simulink model "test_link_demux"  (Simulink 7.3)
settings: Solver=ode45  StartTime=0.0  StopTime=300  RelTol=1e-3
libraries: xbsIndex_r4 x118, xps_library x6, isi_correlator_lib x6, casper_library x2
settings Model: Creator=wjm  LastModifiedBy=wjm
settings OptimizationCC: InitFltsAndDblsToZero=on

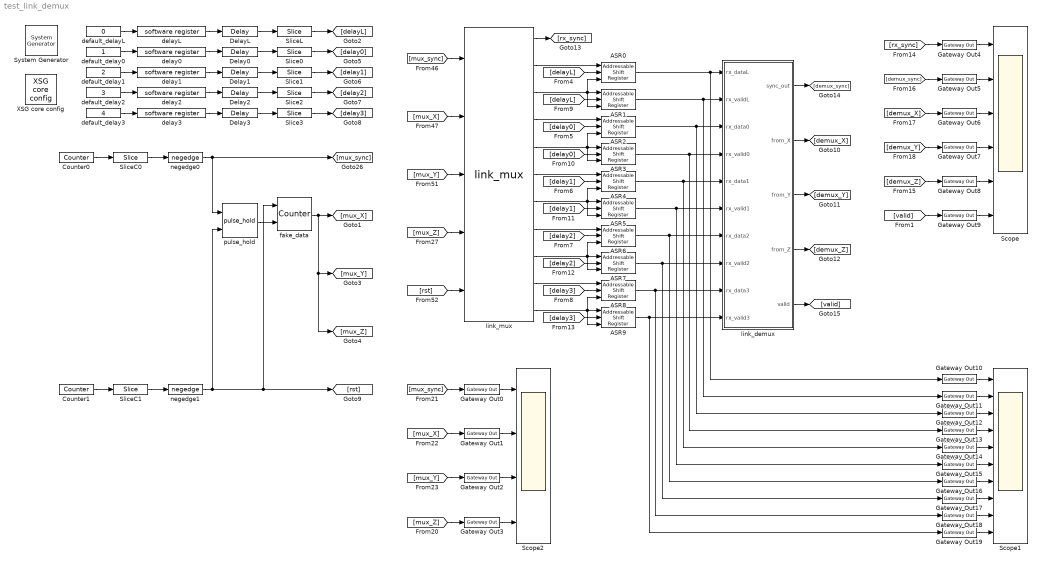
== system test_link_demux ==
  " System Generator" : xbsIndex_r4/ System Generator  Tag=genX  SystemSampleTime=-1  xilinxfamily=virtex5  part=xc5vsx95t  speed=-1  package=ff1136  synthesis_tool=XST  clock_wrapper=Clock Enables  directory=./isi_correlator_cropped/sysgen  testbench=off  simulink_period=1  sysclk_period=5  dcm_input_clock_period=100  incr_netlist=off  trim_vbits=Everywhere in SubSystem  dbl_ovrd=According to Block Masks  core_generation=According to Block Masks  run_coregen=off  deprecated_control=off  eval_field=0  block_type=sysgen
      settings: block_version=10.1.1
  ASR{0..9} (10 alike) : xbsIndex_r4/Addressable Shift Register  infer_latency=on  depth=2  initVector=[0]  en=on  dbl_ovrd=off  use_behavioral_HDL=off  use_rpm=off  block_type=addrsr
      settings: infoedit="Delay of configurable length.  Any element in the delay line can be addressed and driven onto the output port.<br><br>Hardware notes: This block is implemented using SRL16s. If Virtex-4 or Spartan-3 device is used, multiple SRLC16s are cascaded together."  block_version=10.1.3
  Counter0 : xbsIndex_r4/Counter  cnt_type=Free Running  cnt_to=Inf  operation=Up  start_count=2^7-1  cnt_by_val=1  arith_type=Unsigned  n_bits=7  bin_pt=0  load_pin=off  rst=off  en=off  explicit_period=on  period=1  dbl_ovrd=off  use_behavioral_HDL=off  implementation=Fabric  use_rpm=off  block_type=counter
  Counter1 : xbsIndex_r4/Counter  cnt_type=Free Running  cnt_to=Inf  operation=Up  start_count=2^7-1+5  cnt_by_val=1  arith_type=Unsigned  n_bits=9  bin_pt=0  load_pin=off  rst=off  en=off  explicit_period=on  period=1  dbl_ovrd=off  use_behavioral_HDL=off  implementation=Fabric  use_rpm=off  block_type=counter
  Delay{0..3} (4 alike) : xbsIndex_r4/Delay  en=off  latency=3  dbl_ovrd=off  reg_retiming=off  block_type=delay
  DelayL : xbsIndex_r4/Delay  en=off  latency=3  dbl_ovrd=off  reg_retiming=off  block_type=delay
  Gateway Out{0..19} (20 alike) : xbsIndex_r4/Gateway Out  hdl_port=on  timing_constraint=None  locs_specified=off  LOCs={}  block_type=gatewayout
      settings: infoedit="Gateway out block.  Converts Xilinx fixed point inputs into ouputs of type Simulink integer, double, or fixed point.<br><br>Hardware notes:  In hardware these blocks become top level output ports or are discarded, depending on how they are configured."  block_version=11.3
  Scope : Scope  NumInputPorts=6
      settings: TimeRange=150  YMin=0~-1~-1~-1~-1~-1  YMax=1~1~1~1~1~1
  Scope1 : Scope  NumInputPorts=10
      settings: YMin=-5~-5~-5~-5~-5~-5~-5~-5~-5~-5  YMax=5~5~5~5~5~5~5~5~5~5
  Scope2 : Scope  NumInputPorts=4
      settings: YMin=-5~-5~-5~-5  YMax=5~5~5~5  SaveName=ScopeData2
  Slice{0..3} (4 alike) : xbsIndex_r4/Slice  nbits=8  boolean_output=off  mode=Lower Bit Location + Width  bit1=0  base1=MSB of Input  bit0=0  base0=LSB of Input  dbl_ovrd=off  block_type=slice
      settings: block_version=10.1.3
  SliceC0 : xbsIndex_r4/Slice  nbits=1  boolean_output=on  mode=Upper Bit Location + Width  bit1=0  base1=MSB of Input  bit0=0  base0=LSB of Input  dbl_ovrd=off  block_type=slice
      settings: infoedit="Extracts a given range of bits from each input sample and presents it at the output.  The output type is ordinarily unsigned with binary point at zero, but can be Boolean when the slice is one bit wide.<P><P>Hardware notes: In hardware this block costs nothing."  block_version=10.1.3
  SliceC1 : xbsIndex_r4/Slice  nbits=1  boolean_output=on  mode=Upper Bit Location + Width  bit1=0  base1=MSB of Input  bit0=0  base0=LSB of Input  dbl_ovrd=off  block_type=slice
      settings: infoedit="Extracts a given range of bits from each input sample and presents it at the output.  The output type is ordinarily unsigned with binary point at zero, but can be Boolean when the slice is one bit wide.<P><P>Hardware notes: In hardware this block costs nothing."  block_version=10.1.3
  SliceL : xbsIndex_r4/Slice  nbits=8  boolean_output=off  mode=Lower Bit Location + Width  bit1=0  base1=MSB of Input  bit0=0  base0=LSB of Input  dbl_ovrd=off  block_type=slice
      settings: block_version=10.1.3
  XSG core config : xps_library/XSG core config  Tag=xps:xsg  SystemSampleTime=-1  hw_sys=ROACH:sx95t  ibob_linux=off  clk_src=adc0_clk  iBOB_clk_src=sys_clk  BEE2_ctrl_clk_src=sys_clk  BEE2_usr_clk_src=sys_clk  ROACH_clk_src=adc0_clk  CORR_clk_src=sys_clk  gpio_clk_io_group=iBOB:sma  gpio_clk_bit_index=0  clk_rate=200  sample_period=1  synthesis_tool=XST  mpc_type=powerpc440_ext
  default_delay0 : Constant  OutDataType=sfix(16)  OutScaling=2^0  SampleTime=1
  default_delay1 : Constant  Value=2  OutDataType=sfix(16)  OutScaling=2^0  SampleTime=1
  default_delay2 : Constant  Value=3  OutDataType=sfix(16)  OutScaling=2^0  SampleTime=1
  default_delay3 : Constant  Value=4  OutDataType=sfix(16)  OutScaling=2^0  SampleTime=1
  default_delayL : Constant  Value=0  OutDataType=sfix(16)  OutScaling=2^0  SampleTime=1
  delay0 : xps_library/software register  Tag=xps:sw_reg  SystemSampleTime=-1  io_dir=From Processor  arith_type=Unsigned  bitwidth=32  bin_pt=0  sample_period=1  gw_name=test_link_demux_delay0_user_data_out
      link override convert: arith_type=Unsigned  n_bits=32  bin_pt=0
      link override test_link_demux_delay0_user_data_out: arith_type=Unsigned  n_bits=32  bin_pt=0  period=1
  delay1 : xps_library/software register  Tag=xps:sw_reg  SystemSampleTime=-1  io_dir=From Processor  arith_type=Unsigned  bitwidth=32  bin_pt=0  sample_period=1  gw_name=test_link_demux_delay1_user_data_out
      link override convert: arith_type=Unsigned  n_bits=32  bin_pt=0
      link override test_link_demux_delay1_user_data_out: arith_type=Unsigned  n_bits=32  bin_pt=0  period=1
  delay2 : xps_library/software register  Tag=xps:sw_reg  SystemSampleTime=-1  io_dir=From Processor  arith_type=Unsigned  bitwidth=32  bin_pt=0  sample_period=1  gw_name=test_link_demux_delay2_user_data_out
      link override convert: arith_type=Unsigned  n_bits=32  bin_pt=0
      link override test_link_demux_delay2_user_data_out: arith_type=Unsigned  n_bits=32  bin_pt=0  period=1
  delay3 : xps_library/software register  Tag=xps:sw_reg  SystemSampleTime=-1  io_dir=From Processor  arith_type=Unsigned  bitwidth=32  bin_pt=0  sample_period=1  gw_name=test_link_demux_delay3_user_data_out
      link override convert: arith_type=Unsigned  n_bits=32  bin_pt=0
      link override test_link_demux_delay3_user_data_out: arith_type=Unsigned  n_bits=32  bin_pt=0  period=1
  delayL : xps_library/software register  Tag=xps:sw_reg  SystemSampleTime=-1  io_dir=From Processor  arith_type=Unsigned  bitwidth=32  bin_pt=0  sample_period=1  gw_name=test_link_demux_delayL_user_data_out
      link override convert: arith_type=Unsigned  n_bits=32  bin_pt=0
      link override test_link_demux_delayL_user_data_out: arith_type=Unsigned  n_bits=32  bin_pt=0  period=1
  fake_data : xbsIndex_r4/Counter  cnt_type=Free Running  cnt_to=Inf  operation=Up  start_count=0  cnt_by_val=1  arith_type=Unsigned  n_bits=30  bin_pt=0  load_pin=off  rst=on  en=on  explicit_period=on  period=1  dbl_ovrd=off  use_behavioral_HDL=off  implementation=Fabric  use_rpm=off  block_type=counter
  link_demux : Subsystem  AncestorBlock=isi_correlator_lib/link_demux  mask(link_demux){buffer_depth=8, logic_latency=1, mux_latency=1}
      mask prompts: buffer_depth "Buffer depth: (2^n)"; logic_latency "Logic latency:"; mux_latency "Mux latency:"
      mask help: Demuxes three data streams from five links (one loopback and four xaui). Realigns the streams, and reconstructs a corresponding sync pulse.
  link_mux : isi_correlator_lib/link_mux  SystemSampleTime=-1
  negedge0 : casper_library/Misc/negedge  Tag=Rising Edge Detector  SystemSampleTime=-1
  negedge1 : casper_library/Misc/negedge  Tag=Rising Edge Detector  SystemSampleTime=-1
  pulse_hold : isi_correlator_lib/pulse_hold  SystemSampleTime=-1
  wires:
  SliceC0/1 -> negedge0/1
  Counter0/1 -> SliceC0/1
  fake_data/1 -> [mux_Y], [mux_Z], [mux_X]
  SliceC1/1 -> negedge1/1
  Counter1/1 -> SliceC1/1
  negedge0/1 -> pulse_hold/1, [mux_sync]
  negedge1/1 -> pulse_hold/2, fake_data/1, [rst]
  pulse_hold/1 -> fake_data/2
  default_delayL/1 -> delayL/1
  delayL/1 -> DelayL/1
  default_delay0/1 -> delay0/1
  delay0/1 -> Delay0/1
  default_delay1/1 -> delay1/1
  delay1/1 -> Delay1/1
  default_delay2/1 -> delay2/1
  delay2/1 -> Delay2/1
  default_delay3/1 -> delay3/1
  delay3/1 -> Delay3/1
  DelayL/1 -> SliceL/1
  Delay0/1 -> Slice0/1
  Delay1/1 -> Slice1/1
  Delay2/1 -> Slice2/1
  Delay3/1 -> Slice3/1
  ASR0/1 -> link_demux/1(rx_dataL), Gateway Out10/1
  ASR1/1 -> link_demux/2(rx_validL), Gateway Out11/1
  ASR2/1 -> link_demux/3(rx_data0), Gateway Out12/1
  ASR3/1 -> link_demux/4(rx_valid0), Gateway Out13/1
  ASR4/1 -> link_demux/5(rx_data1), Gateway Out14/1
  ASR5/1 -> link_demux/6(rx_valid1), Gateway Out15/1
  ASR6/1 -> link_demux/7(rx_data2), Gateway Out16/1
  ASR7/1 -> link_demux/8(rx_valid2), Gateway Out17/1
  ASR8/1 -> link_demux/9(rx_data3), Gateway Out18/1
  ASR9/1 -> link_demux/10(rx_valid3), Gateway Out19/1
  link_mux/2 -> ASR0/1
  link_mux/3 -> ASR1/1, ASR0/3, ASR1/3
  link_mux/4 -> ASR2/1
  link_mux/5 -> ASR3/1, ASR2/3, ASR3/3
  link_mux/6 -> ASR4/1
  link_mux/7 -> ASR5/1, ASR4/3, ASR5/3
  link_mux/8 -> ASR6/1
  link_mux/9 -> ASR7/1, ASR6/3, ASR7/3
  link_mux/10 -> ASR8/1
  link_mux/11 -> ASR9/1, ASR8/3, ASR9/3
  [mux_sync] -> link_mux/1
  [mux_X] -> link_mux/2
  [mux_Y] -> link_mux/3
  [mux_Z] -> link_mux/4
  [rst] -> link_mux/5
  [delayL] -> ASR0/2
  [delayL] -> ASR1/2
  [delay0] -> ASR2/2
  [delay0] -> ASR3/2
  [delay1] -> ASR4/2
  [delay1] -> ASR5/2
  [delay2] -> ASR6/2
  [delay2] -> ASR7/2
  [delay3] -> ASR8/2
  [delay3] -> ASR9/2
  link_mux/1 -> [rx_sync]
  [rx_sync] -> Gateway Out4/1
  [demux_sync] -> Gateway Out5/1
  [demux_X] -> Gateway Out6/1
  [demux_Y] -> Gateway Out7/1
  [demux_Z] -> Gateway Out8/1
  [mux_sync] -> Gateway Out0/1
  [mux_X] -> Gateway Out1/1
  [mux_Y] -> Gateway Out2/1
  [mux_Z] -> Gateway Out3/1
  link_demux/1(sync_out) -> [demux_sync]
  link_demux/2(from_X) -> [demux_X]
  link_demux/3(from_Y) -> [demux_Y]
  link_demux/4(from_Z) -> [demux_Z]
  link_demux/5(valid) -> [valid]
  SliceL/1 -> [delayL]
  Slice0/1 -> [delay0]
  Slice1/1 -> [delay1]
  Slice2/1 -> [delay2]
  Slice3/1 -> [delay3]
  Gateway Out0/1 -> Scope2/1
  Gateway Out1/1 -> Scope2/2
  Gateway Out2/1 -> Scope2/3
  Gateway Out3/1 -> Scope2/4
  Gateway Out4/1 -> Scope/1
  Gateway Out5/1 -> Scope/2
  Gateway Out6/1 -> Scope/3
  Gateway Out7/1 -> Scope/4
  Gateway Out8/1 -> Scope/5
  Gateway Out10/1 -> Scope1/1
  Gateway Out11/1 -> Scope1/2
  Gateway Out12/1 -> Scope1/3
  Gateway Out13/1 -> Scope1/4
  Gateway Out14/1 -> Scope1/5
  Gateway Out15/1 -> Scope1/6
  Gateway Out16/1 -> Scope1/7
  Gateway Out17/1 -> Scope1/8
  Gateway Out18/1 -> Scope1/9
  Gateway Out19/1 -> Scope1/10
  Gateway Out9/1 -> Scope/6
  [valid] -> Gateway Out9/1

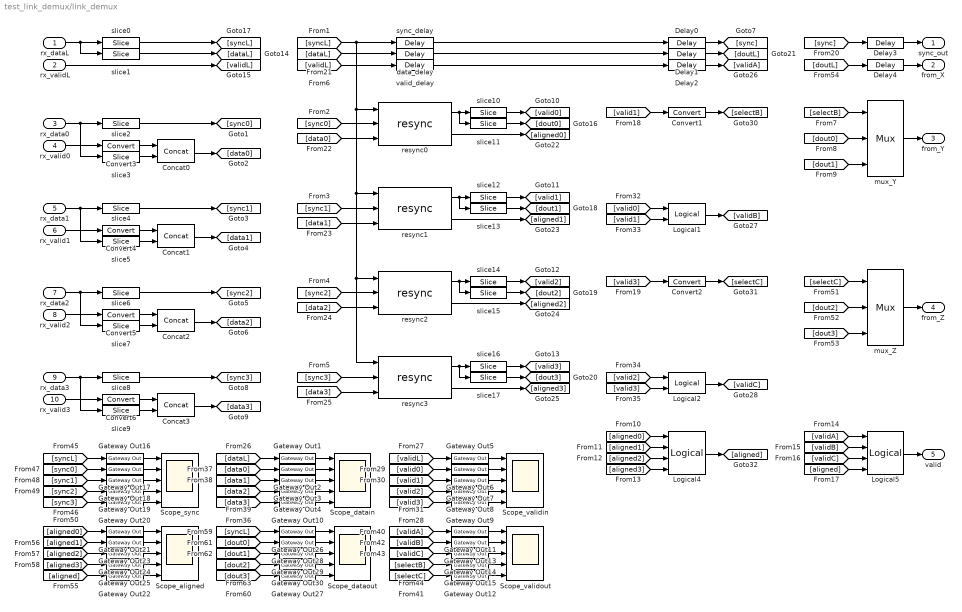
== system test_link_demux/link_demux ==
  rx_dataL : Inport  OutDataType=sfix(16)  OutScaling=2^0
  rx_validL : Inport  Port=2  OutDataType=sfix(16)  OutScaling=2^0
  rx_data0 : Inport  Port=3  OutDataType=sfix(16)  OutScaling=2^0
  rx_valid0 : Inport  Port=4  OutDataType=sfix(16)  OutScaling=2^0
  rx_data1 : Inport  Port=5  OutDataType=sfix(16)  OutScaling=2^0
  rx_valid1 : Inport  Port=6  OutDataType=sfix(16)  OutScaling=2^0
  rx_data2 : Inport  Port=7  OutDataType=sfix(16)  OutScaling=2^0
  rx_valid2 : Inport  Port=8  OutDataType=sfix(16)  OutScaling=2^0
  rx_data3 : Inport  Port=9  OutDataType=sfix(16)  OutScaling=2^0
  rx_valid3 : Inport  Port=10  OutDataType=sfix(16)  OutScaling=2^0
  Concat{0..3} (4 alike) : xbsIndex_r4/Concat  num_inputs=2  dbl_ovrd=off  block_type=concat
      settings: block_version=11.3
  Convert1 : xbsIndex_r4/Convert  arith_type=Unsigned  n_bits=1  bin_pt=0  quantization=Truncate  overflow=Wrap  latency=logic_latency  dbl_ovrd=off  pipeline=off  block_type=convert
      settings: block_version=10.1.3
  Convert2 : xbsIndex_r4/Convert  arith_type=Unsigned  n_bits=1  bin_pt=0  quantization=Truncate  overflow=Wrap  latency=logic_latency  dbl_ovrd=off  pipeline=off  block_type=convert
      settings: block_version=10.1.3
  Convert{3..6} (4 alike) : xbsIndex_r4/Convert  arith_type=Unsigned  n_bits=1  bin_pt=0  quantization=Truncate  overflow=Wrap  latency=0  dbl_ovrd=off  pipeline=off  block_type=convert
      settings: block_version=10.1.3
  Delay0 : xbsIndex_r4/Delay  en=off  latency=logic_latency  dbl_ovrd=off  reg_retiming=off  block_type=delay
  Delay1 : xbsIndex_r4/Delay  en=off  latency=logic_latency  dbl_ovrd=off  reg_retiming=off  block_type=delay
  Delay2 : xbsIndex_r4/Delay  en=off  latency=logic_latency  dbl_ovrd=off  reg_retiming=off  block_type=delay
  Delay3 : xbsIndex_r4/Delay  en=off  latency=mux_latency  dbl_ovrd=off  reg_retiming=off  block_type=delay
  Delay4 : xbsIndex_r4/Delay  en=off  latency=mux_latency  dbl_ovrd=off  reg_retiming=off  block_type=delay
  Gateway Out{1..30} (30 alike) : xbsIndex_r4/Gateway Out  hdl_port=on  timing_constraint=None  locs_specified=off  LOCs={}  block_type=gatewayout
      settings: infoedit="Gateway out block.  Converts Xilinx fixed point inputs into ouputs of type Simulink integer, double, or fixed point.<br><br>Hardware notes:  In hardware these blocks become top level output ports or are discarded, depending on how they are configured."  block_version=11.3
  Logical1 : xbsIndex_r4/Logical  logical_function=XOR  inputs=2  en=off  latency=logic_latency  precision=Full  arith_type=Unsigned  n_bits=16  bin_pt=0  align_bp=on  dbl_ovrd=off  block_type=logical
  Logical2 : xbsIndex_r4/Logical  logical_function=XOR  inputs=2  en=off  latency=logic_latency  precision=Full  arith_type=Unsigned  n_bits=16  bin_pt=0  align_bp=on  dbl_ovrd=off  block_type=logical
  Logical4 : xbsIndex_r4/Logical  logical_function=AND  inputs=4  en=off  latency=logic_latency  precision=Full  arith_type=Unsigned  n_bits=16  bin_pt=0  align_bp=on  dbl_ovrd=off  block_type=logical
  Logical5 : xbsIndex_r4/Logical  logical_function=AND  inputs=4  en=off  latency=mux_latency  precision=Full  arith_type=Unsigned  n_bits=16  bin_pt=0  align_bp=on  dbl_ovrd=off  block_type=logical
  Scope_aligned : Scope  NumInputPorts=5
      settings: TimeRange=300  YMin=0~-1~-1~-1~-1  YMax=1~1~1~1~1  SaveName=ScopeData7
  Scope_datain : Scope  NumInputPorts=5
      settings: TimeRange=300  YMin=0~-1~-1~-1~-1  YMax=1~1~1~1~1  SaveName=ScopeData4
  Scope_dataout : Scope  NumInputPorts=5
      settings: TimeRange=300  YMin=0~-1~-1~-1~-1  YMax=1~1~1~1~1  SaveName=ScopeData8
  Scope_sync : Scope  NumInputPorts=5
      settings: TimeRange=300  YMin=0~-1~-1~-1~-1  YMax=1~1~1~1~1  SaveName=ScopeData6
  Scope_validin : Scope  NumInputPorts=5
      settings: TimeRange=300  YMin=0~-1~-1~-1~-1  YMax=1~1~1~1~1  SaveName=ScopeData3
  Scope_validout : Scope  NumInputPorts=5
      settings: TimeRange=300  YMin=0~-1~-1~-1~-1  YMax=1~1~1~1~1  SaveName=ScopeData5
  data_delay : xbsIndex_r4/Delay  en=off  latency=2^buffer_depth  dbl_ovrd=off  reg_retiming=off  block_type=delay
  mux_Y : xbsIndex_r4/Mux  inputs=2  en=off  latency=mux_latency  precision=Full  arith_type=Unsigned  n_bits=16  bin_pt=14  quantization=Truncate  overflow=Wrap  dbl_ovrd=off  block_type=mux
  mux_Z : xbsIndex_r4/Mux  inputs=2  en=off  latency=mux_latency  precision=Full  arith_type=Unsigned  n_bits=16  bin_pt=14  quantization=Truncate  overflow=Wrap  dbl_ovrd=off  block_type=mux
  resync{0..3} (4 alike) : isi_correlator_lib/resync  SystemSampleTime=-1  depth=buffer_depth
  slice{0,2,4,6,8,10,12,14,16} (9 alike) : xbsIndex_r4/Slice  nbits=1  boolean_output=on  mode=Upper Bit Location + Width  bit1=0  base1=MSB of Input  bit0=0  base0=LSB of Input  dbl_ovrd=off  block_type=slice
      slice0 settings: block_version=10.1.1
      slice10 settings: infoedit="Extracts a given range of bits from each input sample and presents it at the output.  The output type is ordinarily unsigned with binary point at zero, but can be Boolean when the slice is one bit wide.<P><P>Hardware notes: In hardware this block costs nothing."  block_version=10.1.1
      slice12 settings: infoedit="Extracts a given range of bits from each input sample and presents it at the output.  The output type is ordinarily unsigned with binary point at zero, but can be Boolean when the slice is one bit wide.<P><P>Hardware notes: In hardware this block costs nothing."  block_version=10.1.1
      slice14 settings: infoedit="Extracts a given range of bits from each input sample and presents it at the output.  The output type is ordinarily unsigned with binary point at zero, but can be Boolean when the slice is one bit wide.<P><P>Hardware notes: In hardware this block costs nothing."  block_version=10.1.1
      slice16 settings: infoedit="Extracts a given range of bits from each input sample and presents it at the output.  The output type is ordinarily unsigned with binary point at zero, but can be Boolean when the slice is one bit wide.<P><P>Hardware notes: In hardware this block costs nothing."  block_version=10.1.1
      slice2 settings: infoedit="Extracts a given range of bits from each input sample and presents it at the output.  The output type is ordinarily unsigned with binary point at zero, but can be Boolean when the slice is one bit wide.<P><P>Hardware notes: In hardware this block costs nothing."  block_version=10.1.1
      slice4 settings: infoedit="Extracts a given range of bits from each input sample and presents it at the output.  The output type is ordinarily unsigned with binary point at zero, but can be Boolean when the slice is one bit wide.<P><P>Hardware notes: In hardware this block costs nothing."  block_version=10.1.1
      slice6 settings: infoedit="Extracts a given range of bits from each input sample and presents it at the output.  The output type is ordinarily unsigned with binary point at zero, but can be Boolean when the slice is one bit wide.<P><P>Hardware notes: In hardware this block costs nothing."  block_version=10.1.1
      slice8 settings: infoedit="Extracts a given range of bits from each input sample and presents it at the output.  The output type is ordinarily unsigned with binary point at zero, but can be Boolean when the slice is one bit wide.<P><P>Hardware notes: In hardware this block costs nothing."  block_version=10.1.1
  slice{1,11,13,15,17} (5 alike) : xbsIndex_r4/Slice  nbits=30  boolean_output=off  mode=Lower Bit Location + Width  bit1=0  base1=MSB of Input  bit0=0  base0=LSB of Input  dbl_ovrd=off  block_type=slice
      settings: block_version=10.1.1
  slice{3,5,7,9} (4 alike) : xbsIndex_r4/Slice  nbits=31  boolean_output=off  mode=Lower Bit Location + Width  bit1=0  base1=MSB of Input  bit0=0  base0=LSB of Input  dbl_ovrd=off  block_type=slice
      settings: block_version=10.1.1
  sync_delay : xbsIndex_r4/Delay  en=off  latency=2^buffer_depth  dbl_ovrd=off  reg_retiming=off  block_type=delay
  valid_delay : xbsIndex_r4/Delay  en=off  latency=2^buffer_depth  dbl_ovrd=off  reg_retiming=off  block_type=delay
  sync_out : Outport  OutDataType=sfix(16)  OutScaling=2^0
  from_X : Outport  Port=2  OutDataType=sfix(16)  OutScaling=2^0
  from_Y : Outport  Port=3  OutDataType=sfix(16)  OutScaling=2^0
  from_Z : Outport  Port=4  OutDataType=sfix(16)  OutScaling=2^0
  valid : Outport  Port=5  OutDataType=sfix(16)  OutScaling=2^0
  wires:
  Logical5/1 -> valid/1
  Delay3/1 -> sync_out/1
  [sync] -> Delay3/1
  Delay2/1 -> [validA]
  Delay1/1 -> [doutL]
  Delay0/1 -> [sync]
  valid_delay/1 -> Delay2/1
  sync_delay/1 -> Delay0/1
  data_delay/1 -> Delay1/1
  [valid1] -> Convert1/1
  [valid3] -> Convert2/1
  [valid1] -> Logical1/2
  [valid3] -> Logical2/2
  [aligned] -> Logical5/4
  [validC] -> Logical5/3
  [validB] -> Logical5/2
  [validA] -> Logical5/1
  Logical4/1 -> [aligned]
  [aligned3] -> Logical4/4
  [aligned2] -> Logical4/3
  [aligned1] -> Logical4/2
  [aligned0] -> Logical4/1
  Convert1/1 -> [selectB]
  Convert2/1 -> [selectC]
  Logical2/1 -> [validC]
  Logical1/1 -> [validB]
  [validL] -> valid_delay/1
  [valid2] -> Logical2/1
  [valid0] -> Logical1/1
  resync3/2 -> [aligned3]
  slice17/1 -> [dout3]
  slice16/1 -> [valid3]
  resync2/2 -> [aligned2]
  slice15/1 -> [dout2]
  slice14/1 -> [valid2]
  resync1/2 -> [aligned1]
  slice13/1 -> [dout1]
  slice12/1 -> [valid1]
  resync0/2 -> [aligned0]
  slice11/1 -> [dout0]
  slice10/1 -> [valid0]
  resync0/1 -> slice11/1, slice10/1
  resync1/1 -> slice13/1, slice12/1
  resync2/1 -> slice15/1, slice14/1
  resync3/1 -> slice17/1, slice16/1
  [dataL] -> data_delay/1
  [syncL] -> sync_delay/1, resync2/1, resync3/1, resync1/1, resync0/1
  [data3] -> resync3/3
  [sync3] -> resync3/2
  [data2] -> resync2/3
  [sync2] -> resync2/2
  [data1] -> resync1/3
  [sync1] -> resync1/2
  [data0] -> resync0/3
  [sync0] -> resync0/2
  slice8/1 -> [sync3]
  Concat3/1 -> [data3]
  slice6/1 -> [sync2]
  Concat2/1 -> [data2]
  Concat1/1 -> [data1]
  slice4/1 -> [sync1]
  rx_valid3/1 -> Convert6/1
  slice9/1 -> Concat3/2
  rx_valid2/1 -> Convert5/1
  slice7/1 -> Concat2/2
  rx_valid1/1 -> Convert4/1
  slice5/1 -> Concat1/2
  rx_data3/1 -> slice9/1, slice8/1
  rx_data2/1 -> slice7/1, slice6/1
  rx_data1/1 -> slice5/1, slice4/1
  Concat0/1 -> [data0]
  slice3/1 -> Concat0/2
  rx_valid0/1 -> Convert3/1
  slice2/1 -> [sync0]
  rx_data0/1 -> slice3/1, slice2/1
  slice0/1 -> [syncL]
  slice1/1 -> [dataL]
  rx_validL/1 -> [validL]
  rx_dataL/1 -> slice1/1, slice0/1
  Delay4/1 -> from_X/1
  mux_Z/1 -> from_Z/1
  mux_Y/1 -> from_Y/1
  [doutL] -> Delay4/1
  [dout3] -> mux_Z/3
  [dout2] -> mux_Z/2
  [selectC] -> mux_Z/1
  [dout1] -> mux_Y/3
  [dout0] -> mux_Y/2
  [selectB] -> mux_Y/1
  Convert3/1 -> Concat0/1
  Convert4/1 -> Concat1/1
  Convert5/1 -> Concat2/1
  Convert6/1 -> Concat3/1
  [validL] -> Gateway Out5/1
  [valid0] -> Gateway Out6/1
  [valid1] -> Gateway Out7/1
  [valid2] -> Gateway Out8/1
  [valid3] -> Gateway Out9/1
  Gateway Out5/1 -> Scope_validin/1
  Gateway Out6/1 -> Scope_validin/2
  Gateway Out7/1 -> Scope_validin/3
  Gateway Out8/1 -> Scope_validin/4
  Gateway Out9/1 -> Scope_validin/5
  [dataL] -> Gateway Out1/1
  [data0] -> Gateway Out2/1
  [data1] -> Gateway Out3/1
  [data2] -> Gateway Out4/1
  [data3] -> Gateway Out10/1
  Gateway Out1/1 -> Scope_datain/1
  Gateway Out2/1 -> Scope_datain/2
  Gateway Out3/1 -> Scope_datain/3
  Gateway Out4/1 -> Scope_datain/4
  Gateway Out10/1 -> Scope_datain/5
  [validA] -> Gateway Out11/1
  [validB] -> Gateway Out13/1
  [validC] -> Gateway Out14/1
  [selectB] -> Gateway Out15/1
  [selectC] -> Gateway Out12/1
  Gateway Out11/1 -> Scope_validout/1
  Gateway Out13/1 -> Scope_validout/2
  Gateway Out14/1 -> Scope_validout/3
  Gateway Out15/1 -> Scope_validout/4
  Gateway Out12/1 -> Scope_validout/5
  [syncL] -> Gateway Out16/1
  [sync0] -> Gateway Out17/1
  [sync1] -> Gateway Out18/1
  [sync2] -> Gateway Out19/1
  [sync3] -> Gateway Out20/1
  Gateway Out16/1 -> Scope_sync/1
  Gateway Out17/1 -> Scope_sync/2
  Gateway Out18/1 -> Scope_sync/3
  Gateway Out19/1 -> Scope_sync/4
  Gateway Out20/1 -> Scope_sync/5
  [aligned0] -> Gateway Out21/1
  [aligned1] -> Gateway Out23/1
  [aligned2] -> Gateway Out24/1
  [aligned3] -> Gateway Out25/1
  [aligned] -> Gateway Out22/1
  Gateway Out21/1 -> Scope_aligned/1
  Gateway Out23/1 -> Scope_aligned/2
  Gateway Out24/1 -> Scope_aligned/3
  Gateway Out25/1 -> Scope_aligned/4
  Gateway Out22/1 -> Scope_aligned/5
  [syncL] -> Gateway Out26/1
  [dout0] -> Gateway Out28/1
  [dout1] -> Gateway Out29/1
  [dout2] -> Gateway Out30/1
  [dout3] -> Gateway Out27/1
  Gateway Out26/1 -> Scope_dataout/1
  Gateway Out28/1 -> Scope_dataout/2
  Gateway Out29/1 -> Scope_dataout/3
  Gateway Out30/1 -> Scope_dataout/4
  Gateway Out27/1 -> Scope_dataout/5
